simulink model "exercise_3_1"  (R2017a)
settings: Solver=FixedStepAuto  StartTime=0.0  StopTime=simTime  FixedStep=Ts  RelTol=1e-3
values from neighbouring files (symbols this model uses):
  C = Gain*Lead*D*I*I*LP    [exercise_3.m]
  H1 = 1000*((s+6)/(s^3+20*s^2+5000*s))    [exercise_3.m]
libraries: cstblocks x1
settings Model: Creator=marce  LastModifiedBy=marce

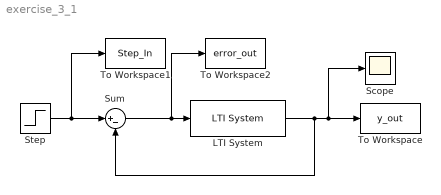
== system exercise_3_1 ==
  LTI System : cstblocks/LTI System  sys=C*H1  IC=[]
  Scope : Scope
  Step : Step  Time=0.1  SampleTime=0
  Sum : Sum  Inputs=|+-
  To Workspace : ToWorkspace  VariableName=y_out  SaveFormat=Timeseries  SampleTime=-1
  To Workspace1 : ToWorkspace  VariableName=Step_In  SaveFormat=Timeseries  SampleTime=-1
  To Workspace2 : ToWorkspace  VariableName=error_out  SaveFormat=Timeseries  SampleTime=-1
  wires:
  Sum/1 -> To Workspace2/1, LTI System/1
  LTI System/1 -> Sum/2, Scope/1, To Workspace/1
  Step/1 -> To Workspace1/1, Sum/1
